simulink model "WashingMachine_esdm"  (R2023a)
settings: Solver=VariableStepAuto  StartTime=0.0  StopTime=10.0  RelTol=1e-3
settings Model: Creator=Simona  LastModifiedBy=Simona

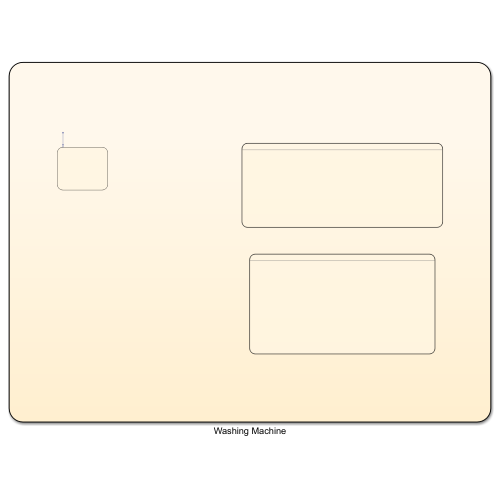
[thumbnail: Simulink's stored preview of the top-level diagram]
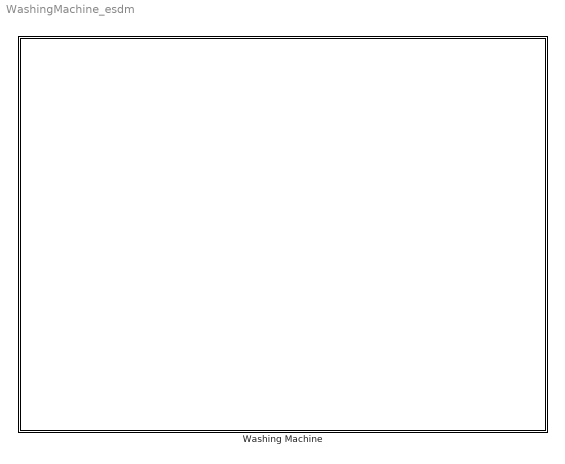
== system WashingMachine_esdm ==
  Washing Machine : Stateflow chart  TreatAsAtomicUnit=on

== stateflow chart WashingMachine_esdm/Washing Machine ==
  state Washing
    state StopFilling
      SpinSpeed=20;
    state Init
      WaterLevel=WaterLevel+1;
      TemperatureLevel=TemperatureLevel+10;
    state Spin
      SpinSpeed==0;
    state Faulty
      MachineStatus==3;
    (default) -> Init
    Init -> StopFilling [order 2] : [WaterLevel==10]
    Spin -> StopFilling : [after(5, sec)]
    StopFilling -> Spin : [after(20,sec)]
    Init -> Faulty [order 1] : [after (160,sec) &&TemperatureLevel<90]
  state IDLE
    du:
    FillWater==0;
    ActivatePump=0;
    HeatWater=0;
    RotatingSpeed=0;
    MachineStatus=0;
  state Rinse
    state InitR
      WaterLevel=WaterLevel-0.9;
    (default) -> InitR : [SpinSpeed==0;]
  (default) -> IDLE : [ProgramSelection==0 || Cancel_button==1 ]
